simulink model "FuelCell_Boost_Controlled"  (R2022b)
settings: Solver=ode45  StartTime=0.0  StopTime=8  RelTol=1e-3  EnableMultiTasking=on
libraries: spsSeriesRLCBranchLib x6, spsIdealSwitchLib x3, spsCurrentMeasurementLib x2, spsDiodeLib x1, spsFuelCellStackLib x1, spsMosfetLib x1, spsPWMGeneratorDCDCLib x1, spsVoltageMeasurementLib x1, sps_lib x1
settings Model: Creator=User  LastModifiedBy=ZinouAb
settings SolverCC: AlgebraicLoopSolver=TrustRegion
settings DataIOCC: LimitDataPoints=on  SaveFormat=Array  SignalLoggingSaveFormat=ModelDataLogs  ReturnWorkspaceOutputs=off
settings OptimizationCC: LifeSpan=inf
settings DebuggingCC: UnderspecifiedInitializationDetection=Classic  MergeDetectMultiDrivingBlocksExec=none  SolverPrmCheckMsg=warning  MultiTaskDSMMsg=warning  MultiTaskCondExecSysMsg=none  UnconnectedInputMsg=warning  UnconnectedOutputMsg=warning  UnconnectedLineMsg=warning  StateNameClashWarn=warning  SFUnexpectedBacktrackingDiag=warning  SFNoUnconditionalDefaultTransitionDiag=warning  SFExecutionAtInitializationDiag=none  SFMachineParentedDataDiag=warning  ArithmeticOperatorsInVariantConditions=warning
settings HardwareCC: ProdBitPerPointer=32  ProdBitPerSizeT=32  ProdBitPerPtrDiffT=32  ProdLargestAtomicFloat=None  ProdIntDivRoundTo=Undefined  ProdEndianess=Unspecified  ProdWordSize=32  ProdHWDeviceType=32-bit Generic
settings ModelReferenceCC: PropagateSignalLabelsOutOfModel=off
settings SFSimCC: SimUseLocalCustomCode=off  CustomCodeUndefinedFunction=UseInterfaceOnly
settings RTWCC: RTWUseLocalCustomCode=off
settings CodeAppCC: StateflowObjectComments=on
settings GRTTargetCC: TargetLangStandard=C89/C90 (ANSI)
settings ConfigComp: CovMetricSettings=dw  CovSaveCumulativeToWorkspaceVar=on  CovSaveSingleToWorkspaceVar=on  CovExternalEMLEnable=off
settings SimscapeCC: SimscapeNormalizeSystem=off

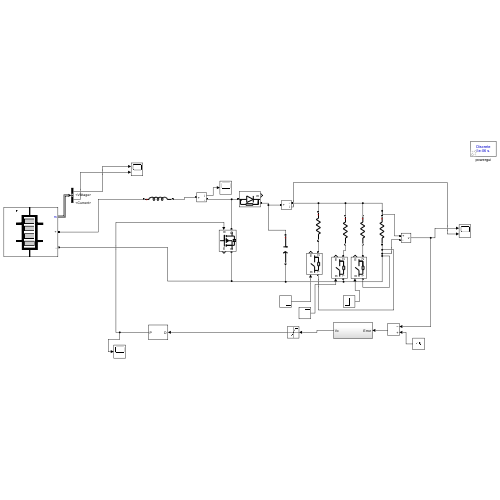
[thumbnail: Simulink's stored preview of the top-level diagram]
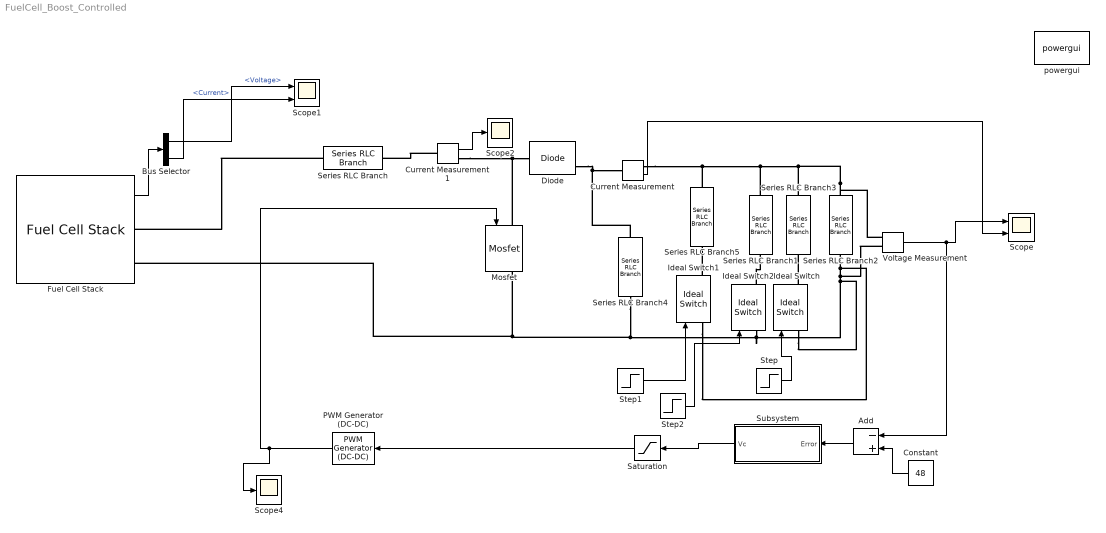
== system FuelCell_Boost_Controlled ==
  Add : Sum  Inputs=-+
  Bus Selector : BusSelector  OutputSignals=Voltage,Current
  Constant : Constant  Value=48
  Current Measurement : spsCurrentMeasurementLib/Current Measurement  PhasorSimulation=off  OutputType=Complex  PSBequivalent=0
  Current Measurement1 : spsCurrentMeasurementLib/Current Measurement  PhasorSimulation=off  OutputType=Complex  PSBequivalent=0
  Diode : spsDiodeLib/Diode  Ron=0.000001  Lon=0  Vf=0  IC=0  UseSnubber=off  Rs=500  Cs=250e-9  Measurements=on
  Fuel Cell Stack : spsFuelCellStackLib/Fuel Cell Stack  PresetModel=PEMFC - 1.26 kW - 24 Vdc  FcType=Proton Exchange Membrane (PEM)  Detailed=Detailed  Eoc=[42,35]  NomVI=[52,24.23]  EndVI=[100,20]  Nc=42  n=46  TOp=55  AirFr=2400  SuppPress=[1.5,1]  Comp=[99.95,21,1]  SignX=off  SignY=off  FlowRateH2=off  FlowRateAir=off  SystemTemp=off  SystemPH2=off  SystemPAir=off  FCDyn=on  FC_tau=0.5  Peak_O2=80  V_Under=10
      settings: LibrarySourceBlock=electricdrivelib/Extra Sources/Fuel Cell Stack
  Ideal Switch : spsIdealSwitchLib/Ideal Switch  Ron=0.00001  Lon=0  IC=0  Rs=1e5  Cs=inf  Measurements=on
  Ideal Switch1 : spsIdealSwitchLib/Ideal Switch  Ron=0.00001  Lon=0  IC=0  Rs=1e5  Cs=inf  Measurements=on
  Ideal Switch2 : spsIdealSwitchLib/Ideal Switch  Ron=0.00001  Lon=0  IC=0  Rs=1e5  Cs=inf  Measurements=on
  Mosfet : spsMosfetLib/Mosfet  Ron=0.1  Lon=0  Rd=0.01  Vfd=0  IC=0  Rs=1e5  Cs=inf  Measurements=on
  PWM Generator (DC-DC) : spsPWMGeneratorDCDCLib/PWM Generator (DC-DC)  Fsw=10000  Ts=0
  Saturation : Saturate  UpperLimit=1  LowerLimit=0
  Scope : Scope  NumInputPorts=2
  Scope1 : Scope  NumInputPorts=2
  Scope2 : Scope
  Scope4 : Scope
  Series RLC Branch : spsSeriesRLCBranchLib/Series RLC Branch  LConnTagsString=__new0  RConnTagsString=__new0  BranchType=L  Resistance=1  Inductance=4.5e-6  SetiL0=on  InitialCurrent=0  Capacitance=1e-6  Setx0=off  InitialVoltage=0  Measurements=None
  Series RLC Branch{1..3,5} (4 alike) : spsSeriesRLCBranchLib/Series RLC Branch  LConnTagsString=__new0  RConnTagsString=__new0  BranchType=R  Resistance=10  Inductance=2e-3  SetiL0=off  InitialCurrent=0  Capacitance=1e-6  Setx0=off  InitialVoltage=0  Measurements=None
  Series RLC Branch4 : spsSeriesRLCBranchLib/Series RLC Branch  LConnTagsString=__new0  RConnTagsString=__new0  BranchType=C  Resistance=100  Inductance=2e-3  SetiL0=off  InitialCurrent=0  Capacitance=900e-5  Setx0=off  InitialVoltage=0  Measurements=None
  Step : Step  Time=4  SampleTime=0
  Step1 : Step  Time=2  Before=1  After=0  SampleTime=0
  Step2 : Step  Time=6  SampleTime=0
  Subsystem : Subsystem
  Voltage Measurement : spsVoltageMeasurementLib/Voltage Measurement  PhasorSimulation=off  OutputType=Complex  PSBequivalent=0
  powergui : sps_lib/powergui  Priority=1  SimulationMode=Discrete  SampleTime=5e-6  frequency=60  Iterations=50  frequencyindice=0  Pbase=100e6  ErrMax=1e-4  UnitsV=kV  UnitsW=MW  buscounter=0  FunctionMessages=off  echomessages=off  EnableUseOfTLC=off  CurrentSourceSwitches=off  DisableSnubberDevices=on  DisableRonSwitches=on  DisableVfSwitches=on  DisplayEquations=off  AutomaticDiscreteSolvers=off  SolverType=Tustin  Interpol=off  ExternalGateDelay=off  methode=off  Ts=0  x0status=blocks  SPID=on  SwTol=0  HookPort=off  NonlinearTolerance=1e-4  nMaxIteration=100  ContinueOnMaxIteration=off  RestoreLinks=warning  ResistiveCurrentMeasurement=off  Frange=[0:2:500]  Ylog=off  Xlog=on  ShowGrid=off  save=off  variable=ZData  structure=0  ZoomFFT=off  StartTime=0.0  cycles=1  DisplayStyle=1  fundamental=60  FreqAxis=off  MaxFrequency=1000  frequencyindicesteady=1  RmsSteady=1  display=off
  wires:
  Voltage Measurement/1 -> Add/1, Scope/1
  Current Measurement/1 -> Scope/2
  Constant/1 -> Add/2
  Add/1 -> Subsystem/1(Error)
  PWM Generator (DC-DC)/1 -> Mosfet/1, Scope4/1
  Saturation/1 -> PWM Generator (DC-DC)/1
  Subsystem/1(Vc) -> Saturation/1
  Fuel Cell Stack/1 -> Bus Selector/1
  Bus Selector/1 -> Scope1/1  "<Voltage>"
  Bus Selector/2 -> Scope1/2  "<Current>"
  Step/1 -> Ideal Switch/1
  Step1/1 -> Ideal Switch1/1
  Step2/1 -> Ideal Switch2/1
  Current Measurement1/1 -> Scope2/1
  connections:
  Mosfet/LConn1 -- Diode/LConn1 -- Current Measurement1/RConn1
  Diode/RConn1 -- Series RLC Branch4/LConn1 -- Current Measurement/LConn1
  Fuel Cell Stack/RConn2 -- Series RLC Branch4/RConn1 -- Ideal Switch/LConn1 -- Voltage Measurement/LConn2 -- Ideal Switch1/LConn1 -- Series RLC Branch2/RConn1 -- Ideal Switch2/LConn1 -- Mosfet/RConn1
  Series RLC Branch/LConn1 -- Fuel Cell Stack/RConn1
  Ideal Switch/RConn1 -- Series RLC Branch3/RConn1
  Ideal Switch1/RConn1 -- Series RLC Branch5/RConn1
  Current Measurement1/LConn1 -- Series RLC Branch/RConn1
  Ideal Switch2/RConn1 -- Series RLC Branch1/RConn1
  Voltage Measurement/LConn1 -- Current Measurement/RConn1 -- Series RLC Branch5/LConn1 -- Series RLC Branch1/LConn1 -- Series RLC Branch3/LConn1 -- Series RLC Branch2/LConn1

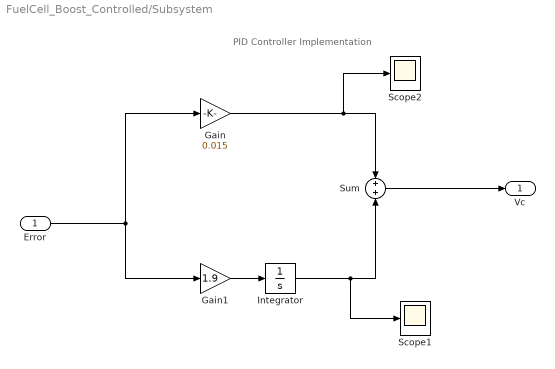
== system FuelCell_Boost_Controlled/Subsystem ==
  note: PID Controller Implementation
  Error : Inport
  Gain : Gain  Gain=0.015
  Gain1 : Gain  Gain=1.9
  Integrator : Integrator  UpperSaturationLimit=0.8  LowerSaturationLimit=0
  Scope1 : Scope
  Scope2 : Scope
  Sum : Sum
  Vc : Outport
  wires:
  Error/1 -> Gain/1, Gain1/1
  Gain1/1 -> Integrator/1
  Gain/1 -> Scope2/1, Sum/1
  Sum/1 -> Vc/1
  Integrator/1 -> Scope1/1, Sum/2
